simulink model "untitled1xzvz"  (Simulink 7.5)
settings: Solver=ode45  StartTime=0.0  StopTime=10.0  RelTol=1e-3
libraries: powerlib x5
settings Model: Creator=dell  LastModifiedBy=dell

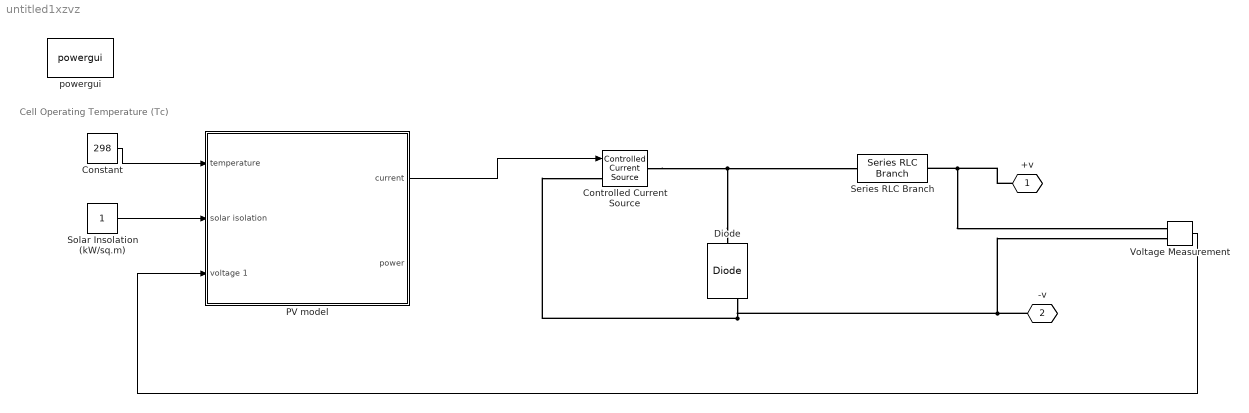
== system untitled1xzvz ==
  note: Cell Operating Temperature (Tc)
  Constant : Constant  Value=298  VectorParams1D=off  OutDataType=fixdt(1, 16)  OutScaling=2^0
  Controlled Current Source : powerlib/Electrical Sources/Controlled Current Source  DialogController=POWERSYS.PowerSysDialog  SystemSampleTime=-1  Initialize=on  Source_Type=DC  Amplitude=0  Phase=0  Frequency=0  Measurements=Current
  Diode : powerlib/Power Electronics/Diode  DialogController=POWERSYS.PowerSysDialog  SystemSampleTime=-1  Ron=0.001  Lon=0  Vf=0.8  IC=0  UseSnubber=off  Rs=500  Cs=250e-9  Measurements=on
  PV model : Subsystem
  Series RLC Branch : powerlib/Elements/Series RLC Branch  DialogController=POWERSYS.PowerSysDialog  PhysicalDomain=powersysdomain  SubClassName=unknown  LeftPortType=p1  RightPortType=p1  LConnTagsString=__new0  RConnTagsString=__new0  BranchType=R  Resistance=0.001  Inductance=1e-3  SetiL0=off  InitialCurrent=0  Capacitance=1e-6  Setx0=off  InitialVoltage=0  Measurements=None
  Solar Insolation (kW/sq.m) : Constant  OutDataType=fixdt(1, 16)  OutScaling=2^0
  Voltage Measurement : powerlib/Measurements/Voltage Measurement  DialogController=POWERSYS.PowerSysDialog  SystemSampleTime=-1  PhasorSimulation=off  OutputType=Complex  PSBequivalent=0
  powergui : powerlib/powergui  Priority=1  SystemSampleTime=-1  SimulationMode=Continuous  SampleTime=50e-6  frequency=60  SPID=off  DisableSnubberDevices=off  DisableRonSwitches=off  DisableVfSwitches=off  SwTol=0  Interpol=off  frequencyindice=0  echomessages=off  HookPort=off  DisplayEquations=off  FunctionMessages=off  EnableUseOfTLC=off  x0status=blocks  RestoreLinks=warning  ResistiveCurrentMeasurement=off  Ylog=off  Xlog=on  ShowGrid=off  save=off  variable=ZData  ZoomFFT=off  StartTime=0.0  cycles=1  DisplayStyle=1  FreqAxis=off  MaxFrequency=1000  frequencyindicesteady=1  display=off  methode=off
  +v : PMIOPort  Tag=PMCPort  Port=1  Side=Left
  -v : PMIOPort  Tag=PMCPort  Port=2  Side=Right
  wires:
  Constant/1 -> PV model/1(temperature)
  Solar Insolation (kW/sq.m)/1 -> PV model/2(solar isolation)
  PV model/1(current) -> Controlled Current Source/1
  Voltage Measurement/1 -> PV model/3(voltage 1)
  connections:
  Diode/LConn1 -- Controlled Current Source/RConn1 -- Series RLC Branch/LConn1
  Diode/RConn1 -- -v/RConn1 -- Voltage Measurement/LConn2 -- Controlled Current Source/LConn1
  +v/RConn1 -- Series RLC Branch/RConn1 -- Voltage Measurement/LConn1

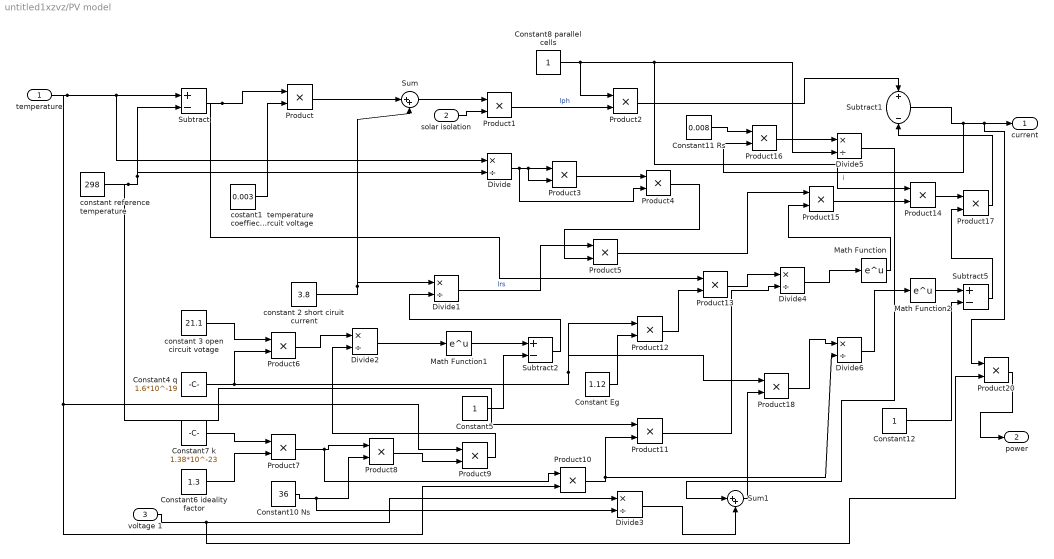
== system untitled1xzvz/PV model ==
  temperature : Inport  OutDataType=fixdt(1, 16)  OutScaling=2^0
  solar isolation : Inport  Port=2  OutDataType=fixdt(1, 16)  OutScaling=2^0
  voltage 1 : Inport  Port=3  OutDataType=fixdt(1, 16)  OutScaling=2^0
  Constant Eg : Constant  Value=1.12  OutDataType=fixdt(1, 16)  OutScaling=2^0
  Constant10 Ns : Constant  Value=36  OutDataType=fixdt(1, 16)  OutScaling=2^0
  Constant11 Rs : Constant  Value=0.008  OutDataType=fixdt(1, 16)  OutScaling=2^0
  Constant12 : Constant  OutDataType=fixdt(1, 16)  OutScaling=2^0
  Constant4 q : Constant  Value=1.6*10^-19  OutDataType=fixdt(1, 16)  OutScaling=2^0
  Constant5 : Constant  OutDataType=fixdt(1, 16)  OutScaling=2^0
  Constant6 ideality factor : Constant  Value=1.3  OutDataType=fixdt(1, 16)  OutScaling=2^0
  Constant7 k : Constant  Value=1.38*10^-23  OutDataType=fixdt(1, 16)  OutScaling=2^0
  Constant8 parallel cells : Constant  OutDataType=fixdt(1, 16)  OutScaling=2^0
  Divide{,1..6} (7 alike) : Product  Inputs=*/  OutDataType=fixdt(1, 16)  OutScaling=2^-10
  Math Function : Math  OutDataType=fixdt(1, 16)  OutScaling=2^0  SaturateOnIntegerOverflow=on
  Math Function1 : Math  OutDataType=fixdt(1, 16)  OutScaling=2^0  SaturateOnIntegerOverflow=on
  Math Function2 : Math  OutDataType=fixdt(1, 16)  OutScaling=2^0  SaturateOnIntegerOverflow=on
  Product{,1..18,20} (20 alike) : Product  OutDataType=fixdt(1, 16)  OutScaling=2^0  RndMeth=Zero
  Subtract{,1..2,5} (4 alike) : Sum  Inputs=+-  OutDataType=fixdt(1, 16)  OutScaling=2^-10
  Sum : Sum  Inputs=|++  OutDataType=fixdt(1, 16)  OutScaling=2^0
  Sum1 : Sum  Inputs=|++  OutDataType=fixdt(1, 16)  OutScaling=2^0
  constant 2 short ciruit current : Constant  Value=3.8  OutDataType=fixdt(1, 16)  OutScaling=2^0
  constant 3 open circuit votage : Constant  Value=21.1  OutDataType=fixdt(1, 16)  OutScaling=2^0
  constant reference temperature : Constant  Value=298  OutDataType=fixdt(1, 16)  OutScaling=2^0
  costant1  temperature coeffiecent of open circuit voltage : Constant  Value=0.003  OutDataType=fixdt(1, 16)  OutScaling=2^0
  current : Outport  OutDataType=fixdt(1, 16)  OutScaling=2^0
  power : Outport  Port=2  OutDataType=fixdt(1, 16)  OutScaling=2^0
  wires:
  temperature/1 -> Subtract/1, Divide/1, Product10/2, Product9/1
  costant1  temperature coeffiecent of open circuit voltage/1 -> Product/2
  constant reference temperature/1 -> Subtract/2, Divide/2, Product11/1
  Subtract/1 -> Product/1, Product13/1
  Product/1 -> Sum/1
  constant 2 short ciruit current/1 -> Sum/2, Divide1/1
  Sum/1 -> Product1/1
  solar isolation/1 -> Product1/2
  Product1/1 -> Product2/2  "Iph"
  Constant8 parallel cells/1 -> Product2/1, Divide5/2, Product14/1
  Product2/1 -> Subtract1/1
  Divide/1 -> Product3/1, Product3/2, Product4/2
  Product3/1 -> Product4/1
  Product4/1 -> Product5/2
  Divide1/1 -> Product5/1  "Irs"
  constant 3 open circuit votage/1 -> Product6/1
  Constant4 q/1 -> Product6/2, Product12/1, Product18/1
  Product6/1 -> Divide2/1
  Divide2/1 -> Math Function1/1
  Math Function1/1 -> Subtract2/1
  Subtract2/1 -> Divide1/2
  Constant5/1 -> Subtract2/2
  Constant7 k/1 -> Product7/1
  Constant6 ideality factor/1 -> Product7/2
  Product7/1 -> Product8/1, Product10/1
  Constant10 Ns/1 -> Product8/2, Divide3/2
  Product8/1 -> Product9/2
  Product9/1 -> Divide2/2
  Product10/1 -> Product11/2, Divide6/2
  voltage 1/1 -> Divide3/1, Product20/2
  Constant Eg/1 -> Product12/2
  Product12/1 -> Product13/2
  Product13/1 -> Divide4/1
  Divide4/1 -> Math Function/1
  Math Function/1 -> Product15/2
  Product5/1 -> Product15/1
  Constant11 Rs/1 -> Product16/1
  Product16/1 -> Divide5/1
  Subtract1/1 -> Product16/2, Product20/1, current/1  "i"
  Product15/1 -> Product14/2
  Product17/1 -> Subtract1/2
  Product14/1 -> Product17/1
  Math Function2/1 -> Subtract5/1
  Subtract5/1 -> Product17/2
  Divide6/1 -> Math Function2/1
  Constant12/1 -> Subtract5/2
  Product18/1 -> Divide6/1
  Product11/1 -> Divide4/2
  Divide3/1 -> Sum1/2
  Divide5/1 -> Sum1/1
  Sum1/1 -> Product18/2
  Product20/1 -> power/1
